simulink model "mpc_customQPcodegen"  (R2023a)
settings: Solver=FixedStepAuto  StartTime=0.0  StopTime=7  MaxStep=0.1  MinStep=0.01  RelTol=1e-3  EnableMultiTasking=on
undefined symbols (not defined in the file or in its folder): tau
libraries: cstblocks x1, mpclib x1
settings Model: Creator=The MathWorks, Inc.  LastModifiedBy=The MathWorks, Inc.
settings SolverCC: AlgebraicLoopSolver=TrustRegion  MinimalZcImpactIntegration=on
settings DataIOCC: LimitDataPoints=on  SaveFormat=Array  ReturnWorkspaceOutputs=off
settings OptimizationCC: ExpressionDepthLimit=2147483647  LifeSpan=inf
settings DebuggingCC: UnderspecifiedInitializationDetection=Classic  MergeDetectMultiDrivingBlocksExec=none  SolverPrmCheckMsg=warning  FcnCallInpInsideContextMsg=warning  UnconnectedInputMsg=warning  UnconnectedOutputMsg=warning  UnconnectedLineMsg=warning  StateNameClashWarn=warning  SFUnexpectedBacktrackingDiag=warning  SFNoUnconditionalDefaultTransitionDiag=warning  SFExecutionAtInitializationDiag=none  ArithmeticOperatorsInVariantConditions=warning
settings HardwareCC: ProdBitPerPointer=32  ProdBitPerSizeT=32  ProdBitPerPtrDiffT=32  ProdLargestAtomicFloat=None  ProdIntDivRoundTo=Undefined  ProdEndianess=Unspecified  ProdWordSize=32  ProdHWDeviceType=32-bit Generic
settings ModelReferenceCC: EnableRefExpFcnMdlSchedulingChecks=on  PropagateSignalLabelsOutOfModel=off
settings SFSimCC: SimUseLocalCustomCode=off  CustomCodeUndefinedFunction=UseInterfaceOnly
settings RTWCC: RTWVerbose=off  RTWUseLocalCustomCode=off
settings CodeAppCC: StateflowObjectComments=on
settings GRTTargetCC: TargetLangStandard=C89/C90 (ANSI)  CombineOutputUpdateFcns=off  GRTInterface=on
settings ConfigComp: CovMetricSettings=dw  CovSaveCumulativeToWorkspaceVar=on  CovSaveSingleToWorkspaceVar=on  CovExternalEMLEnable=off  CovSFcnEnable=off

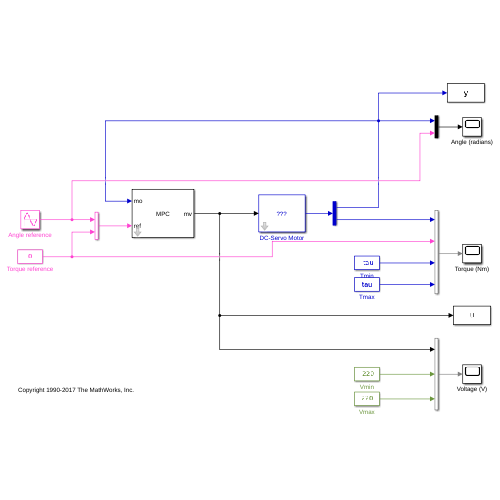
[thumbnail: Simulink's stored preview of the top-level diagram]
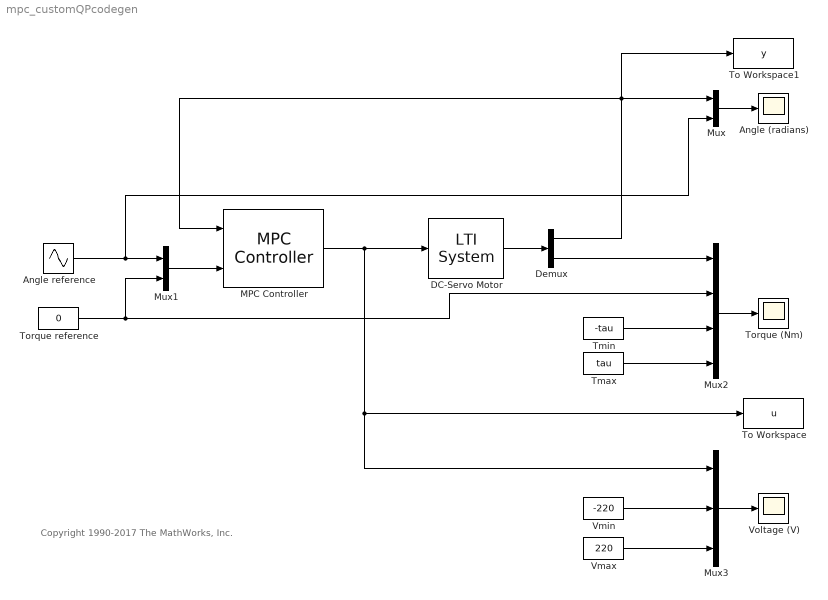
== system mpc_customQPcodegen ==
  note: Copyright 1990-2017 The MathWorks, Inc.
  Angle (radians) : Scope
  Angle reference : Sin  Amplitude=pi  Frequency=.4  SampleTime=0
  DC-Servo Motor : cstblocks/LTI System  sys=plant  IC=[]
  Demux : Demux  Outputs=2
      settings: DisplayOption=none
  MPC Controller : mpclib/MPC Controller  mpcobj=mpcobj  x0=[]  is_multiple=0  enable_value=0  return_u0=off  updateMPCinCallerWorkspace=on  md_inport=off  mv_inport=off  uref_inport=off  return_cost=off  return_mvseq=off  return_qpstatus=off  return_xseq=off  return_state=off  return_ovseq=off  state_inport=off  umin_inport=off  umax_inport=off  ymin_inport=off  ymax_inport=off  cc_inport=off  ywt_inport=off  uwt_inport=off  duwt_inport=off  rhoeps_inport=off  pm_inport=off  MaximumP=10  HorizonChoice=FixedHorizon  n_ts=0.1  n_p=10  n_mv=1  n_md=0  n_ud=0  n_mo=1  n_uo=1  BlockDataType=double  SampleTimeInherited=off  switch_inport=off
  Mux : Mux  Inputs=2
  Mux1 : Mux  Inputs=2
  Mux2 : Mux
  Mux3 : Mux  Inputs=3
  Tmax : Constant  Value=tau
  Tmin : Constant  Value=-tau
  To Workspace : ToWorkspace  VariableName=u  SaveFormat=Structure With Time  SampleTime=-1
  To Workspace1 : ToWorkspace  VariableName=y  SaveFormat=Structure With Time  SampleTime=-1
  Torque (Nm) : Scope
  Torque reference : Constant  Value=0
  Vmax : Constant  Value=220
  Vmin : Constant  Value=-220
  Voltage (V) : Scope
  wires:
  Mux1/1 -> MPC Controller/2
  Tmin/1 -> Mux2/3
  Tmax/1 -> Mux2/4
  Vmax/1 -> Mux3/3
  Vmin/1 -> Mux3/2
  Mux3/1 -> Voltage (V)/1
  Angle reference/1 -> Mux/2, Mux1/1
  Demux/2 -> Mux2/1
  Mux2/1 -> Torque (Nm)/1
  Torque reference/1 -> Mux1/2, Mux2/2
  Mux/1 -> Angle (radians)/1
  DC-Servo Motor/1 -> Demux/1
  MPC Controller/1 -> Mux3/1, To Workspace/1, DC-Servo Motor/1
  Demux/1 -> To Workspace1/1, MPC Controller/1, Mux/1
